simulink model "crazyflie"  (R2020b)
settings: Solver=FixedStepDiscrete  StartTime=0.0  StopTime=160  FixedStep=0.0001  RelTol=1e-3
values from neighbouring files (symbols this model uses):
  g = 9.81    [linearized_states.m]
  Ts = 0.0001    [linearized_states.m]
undefined symbols (not defined in the file or in its folder): K
settings Model: PauseTimes=7  Creator=Zrean  LastModifiedBy=carle
settings DataIOCC: ReturnWorkspaceOutputs=off
settings OptimizationCC: DefaultParameterBehavior=Inlined  UseDivisionForNetSlopeComputation=on  UseFloatMulNetSlope=on  UseSpecifiedMinMax=on  InlineInvariantSignals=on  PassReuseOutputArgsAs=Individual arguments  ZeroExternalMemoryAtStartup=off  ZeroInternalMemoryAtStartup=off  NoFixptDivByZeroProtection=on  EfficientFloat2IntCast=on  LifeSpan=1  EfficientTunableParamExpr=on
settings DebuggingCC: AlgebraicLoopMsg=error  ParameterTunabilityLossMsg=error  ArithmeticOperatorsInVariantConditions=warning
settings HardwareCC: ProdBitPerPointer=32  ProdBitPerSizeT=32  ProdBitPerPtrDiffT=32  ProdLargestAtomicInteger=Long  ProdLargestAtomicFloat=Double  ProdWordSize=32  ProdHWDeviceType=ARM Compatible->ARM Cortex
settings SFSimCC: SimUseLocalCustomCode=off  MATLABDynamicMemAlloc=off  CustomCodeUndefinedFunction=UseInterfaceOnly
settings RTWCC: Description=Embedded Coder  SystemTargetFile=ert.tlc  GenCodeOnly=on  TemplateMakefile=ert_default_tmf  GenerateReport=on  RTWUseLocalCustomCode=off  BuildConfiguration=Faster Runs  IncludeHyperlinkInReport=on  LaunchReport=on  GenerateTraceInfo=on  GenerateTraceReport=on  GenerateTraceReportSl=on  GenerateTraceReportSf=on  GenerateTraceReportEml=on  GenerateCodeMetricsReport=on
settings CodeAppCC: ForceParamTrailComments=on  IgnoreCustomStorageClasses=off  OperatorAnnotations=on  SimulinkDataObjDesc=on  SFDataObjDesc=on  MATLABFcnDesc=on  InsertBlockDesc=on  StateflowObjectComments=on  MATLABSourceComments=on
settings ERTTargetCC: TargetLangStandard=C99 (ISO)  MultiwordLength=2048  CombineSignalStateStructs=on  SuppressErrorStatus=on  SupportAbsoluteTime=off  SupportNonFinite=off  SupportComplex=off  InlinedParameterPlacement=NonHierarchical  ERTCustomFileTemplate=crazyflie_wrapper.tlc  ERTFilePackagingFormat=CompactWithDataFile
settings SimscapeCC: SimscapeNormalizeSystem=off

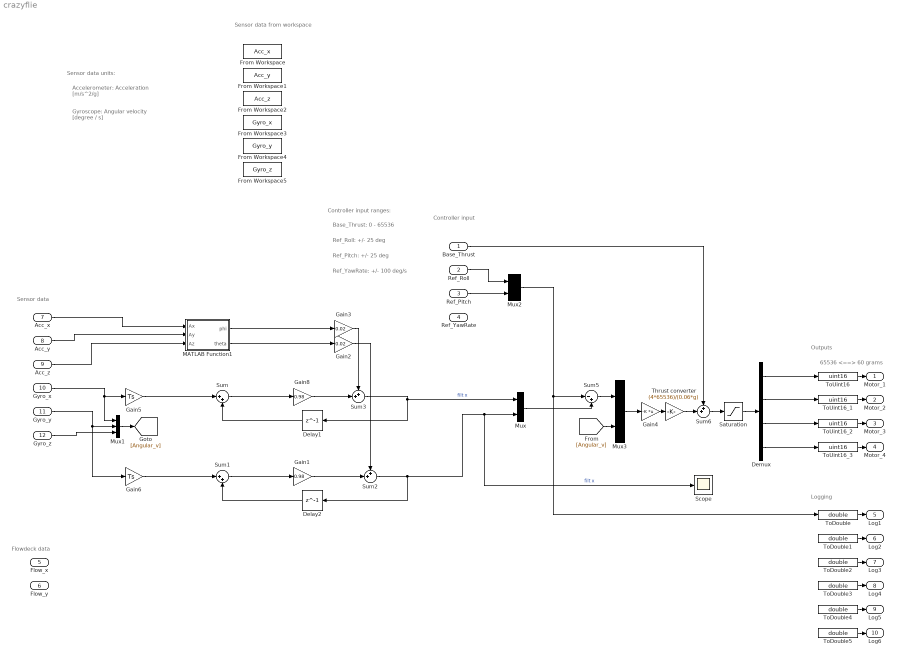
== system crazyflie ==
  note: 65536 <==> 60 grams
  note: Logging
  note: Outputs
  note: Controller input
  note: Ref_Roll: +/- 25 deg
  note: Base_Thrust: 0 - 65536
  note: Ref_Pitch: +/- 25 deg
  note: Ref_YawRate: +/- 100 deg/s
  note: Controller input ranges:
  note: Gyroscope:
      | Angular velocity [degree / s]
  note: Accelerometer:
      | Acceleration [m/s^2/g]
  note: Sensor data units:
  note: Flowdeck data
  note: Sensor data
  note: Sensor data from
      | workspace
  Base_Thrust : Inport  OutDataTypeStr=double
  Ref_Roll : Inport  Port=2  OutDataTypeStr=double
  Ref_Pitch : Inport  Port=3  OutDataTypeStr=double
  Ref_YawRate : Inport  Port=4  OutDataTypeStr=double
  Flow_x : Inport  Port=5  OutDataTypeStr=int16  PortDimensions=1
  Flow_y : Inport  Port=6  OutDataTypeStr=int16  PortDimensions=1
  Acc_x : Inport  Port=7  OutDataTypeStr=double  PortDimensions=1
  Acc_y : Inport  Port=8  OutDataTypeStr=double  PortDimensions=1
  Acc_z : Inport  Port=9  OutDataTypeStr=double  PortDimensions=1
  Gyro_x : Inport  Port=10  OutDataTypeStr=double  PortDimensions=1
  Gyro_y : Inport  Port=11  OutDataTypeStr=double  PortDimensions=1
  Gyro_z : Inport  Port=12  OutDataTypeStr=double  PortDimensions=1
  Delay1 : Delay  DelayLength=1  InitialCondition=0
  Delay2 : Delay  DelayLength=1  InitialCondition=0
  Demux : Demux
  From Workspace : FromWorkspace  VariableName=Acc_x  OutDataTypeStr=double
  From Workspace1 : FromWorkspace  VariableName=Acc_y  OutDataTypeStr=double
  From Workspace2 : FromWorkspace  VariableName=Acc_z  OutDataTypeStr=double
  From Workspace3 : FromWorkspace  VariableName=Gyro_x  OutDataTypeStr=double
  From Workspace4 : FromWorkspace  VariableName=Gyro_y  OutDataTypeStr=double
  From Workspace5 : FromWorkspace  VariableName=Gyro_z  OutDataTypeStr=double
  Gain1 : Gain  Gain=0.98
  Gain2 : Gain  Gain=0.02
  Gain3 : Gain  Gain=0.02
  Gain4 : Gain  Gain=-K  Multiplication=Matrix(K*u)
  Gain5 : Gain  Gain=Ts
  Gain6 : Gain  Gain=Ts
  Gain8 : Gain  Gain=0.98
  MATLAB Function1 : MATLAB Function  TreatAsAtomicUnit=on
  Mux : Mux  Inputs=2
  Mux1 : Mux  Inputs=3
  Mux2 : Mux  Inputs=2
  Mux3 : Mux  Inputs=2
  Saturation : Saturate  UpperLimit=65536  LowerLimit=0
  Scope : Scope
  Sum : Sum  Inputs=|++
  Sum1 : Sum  Inputs=|++
  Sum2 : Sum  Inputs=++|
  Sum3 : Sum  Inputs=++|
  Sum5 : Sum  Inputs=|-+
  Sum6 : Sum  Inputs=++|
  Thrust converter : Gain  Gain=(4*65536)/(0.06*g)
  ToDouble{,1..5} (6 alike) : DataTypeConversion  OutDataTypeStr=double  SaturateOnIntegerOverflow=on
  ToUint16 : DataTypeConversion  OutDataTypeStr=uint16  SaturateOnIntegerOverflow=on
  ToUint16_1 : DataTypeConversion  OutDataTypeStr=uint16  SaturateOnIntegerOverflow=on
  ToUint16_2 : DataTypeConversion  OutDataTypeStr=uint16  SaturateOnIntegerOverflow=on
  ToUint16_3 : DataTypeConversion  OutDataTypeStr=uint16  SaturateOnIntegerOverflow=on
  Motor_1 : Outport  OutDataTypeStr=uint16  VectorParamsAs1DForOutWhenUnconnected=off  LockScale=on
  Motor_2 : Outport  Port=2  OutDataTypeStr=uint16  VectorParamsAs1DForOutWhenUnconnected=off  LockScale=on
  Motor_3 : Outport  Port=3  OutDataTypeStr=uint16  VectorParamsAs1DForOutWhenUnconnected=off  LockScale=on
  Motor_4 : Outport  Port=4  OutDataTypeStr=uint16  VectorParamsAs1DForOutWhenUnconnected=off  LockScale=on
  Log1 : Outport  Port=5  OutDataTypeStr=double  VectorParamsAs1DForOutWhenUnconnected=off
  Log2 : Outport  Port=6  OutDataTypeStr=double  VectorParamsAs1DForOutWhenUnconnected=off
  Log3 : Outport  Port=7  OutDataTypeStr=double  VectorParamsAs1DForOutWhenUnconnected=off
  Log4 : Outport  Port=8  OutDataTypeStr=double  VectorParamsAs1DForOutWhenUnconnected=off
  Log5 : Outport  Port=9  OutDataTypeStr=double  VectorParamsAs1DForOutWhenUnconnected=off
  Log6 : Outport  Port=10  OutDataTypeStr=double  VectorParamsAs1DForOutWhenUnconnected=off
  wires:
  ToUint16/1 -> Motor_1/1
  ToUint16_1/1 -> Motor_2/1
  ToUint16_2/1 -> Motor_3/1
  ToUint16_3/1 -> Motor_4/1
  ToDouble/1 -> Log1/1
  ToDouble1/1 -> Log2/1
  ToDouble2/1 -> Log3/1
  ToDouble3/1 -> Log4/1
  ToDouble4/1 -> Log5/1
  ToDouble5/1 -> Log6/1
  Gain5/1 -> Sum/1
  Delay1/1 -> Sum/2
  Gain8/1 -> Sum3/2
  Sum/1 -> Gain8/1
  Acc_x/1 -> MATLAB Function1/1(Ax)
  Acc_z/1 -> MATLAB Function1/3(Az)
  Gyro_x/1 -> Mux1/1, Gain5/1
  Gyro_y/1 -> Mux1/2, Gain6/1
  Gain3/1 -> Sum3/1
  Sum3/1 -> Delay1/1, Mux/1  "filt x"
  Sum1/1 -> Gain1/1
  Gain1/1 -> Sum2/2
  Delay2/1 -> Sum1/2
  Gain6/1 -> Sum1/1
  Sum2/1 -> Scope/1, Mux/2, Delay2/1  "filt x"
  Gain2/1 -> Sum2/1
  Mux1/1 -> [Angular_v]
  Gyro_z/1 -> Mux1/3
  Ref_Roll/1 -> Mux2/1
  Ref_Pitch/1 -> Mux2/2
  Mux/1 -> Sum5/2
  Sum5/1 -> Mux3/1
  [Angular_v] -> Mux3/2
  Mux3/1 -> Gain4/1
  Sum6/1 -> Saturation/1
  Saturation/1 -> Demux/1
  Demux/2 -> ToUint16_1/1
  Demux/3 -> ToUint16_2/1
  Demux/4 -> ToUint16_3/1
  Demux/1 -> ToUint16/1
  Acc_y/1 -> MATLAB Function1/2(Ay)
  MATLAB Function1/2(theta) -> Gain2/1
  MATLAB Function1/1(phi) -> Gain3/1
  Mux2/1 -> ToDouble/1, Sum5/1
  Gain4/1 -> Thrust converter/1
  Base_Thrust/1 -> Sum6/1
  Thrust converter/1 -> Sum6/2

== matlab function crazyflie/MATLAB Function1 ==
  data: phi output; Ax input; theta output; Ay input; Az input
function [phi, theta] = fcn(Ax,Ay,Az)
    
phi = atan2d(Ay,Az);
theta = atan2d(-Ax,norm([Ay Az]));
end
